simulink model "lab5_friccomp"  (Simulink 8.9)
settings: Solver=ode1  StartTime=0.0  StopTime=10  FixedStep=0.002  RelTol=1e-3  EnableMultiTasking=on
libraries: simulink x2, coecsllib x1, fricblocks x1
Description:
  | Real-Time Van der Pol Simulation
  | 
  | This demonstration shows a real-time version of the Simulink(R) Van der Pol
  | simulation demo. This model does not need any external signals, so it does
  | not need any data acquisition hardware or driver. This makes the model ideal
  | for first experiments with Real-Time Windows Target(TM), without need to
  | worry about proper I/O hardware configuration.
  | 
  | How to run this demo:
  | 
  |   1. Build the model using Tools -> Real-Time Workshop -> Build Model.
  |   2. Connect to the real-time code using Simulation -> Connect to target.
  |   3. Start the real-time execution using Simulation -> Start real-time code.
settings Model: Creator=Houska  LastModifiedBy=maherna4  SimulationMode=external  ExtModeTrigDuration=50000
settings DataIOCC: SignalLoggingName=logsOut
settings OptimizationCC: ExpressionDepthLimit=2147483647  InitFltsAndDblsToZero=on  EfficientMapNaN2IntZero=off  LifeSpan=auto
settings DebuggingCC: SignalResolutionControl=TryResolveAllWithWarning
settings HardwareCC: ProdBitPerPointer=64  ProdBitPerSizeT=64  ProdBitPerPtrDiffT=64  ProdLargestAtomicFloat=Float  ProdIntDivRoundTo=Zero  ProdEndianess=LittleEndian  ProdWordSize=64  ProdHWDeviceType=Intel->x86-64 (Windows64)  TargetBitPerLong=64  TargetBitPerPointer=64  TargetIntDivRoundTo=Zero  TargetEndianess=LittleEndian  TargetWordSize=64  TargetHWDeviceType=Intel->x86-64
settings RTWCC: SystemTargetFile=sldrt.tlc  TemplateMakefile=sldrt.tmf  Description=Simulink Desktop Real-Time  RTWCompilerOptimization=on
settings CodeAppCC: MaxIdLength=95
settings SimulinkDesktopRealTimeCC: TargetPreCompLibLocation=C:\MATLABR2017a\toolbox\sldrt\lib\win64  TargetLangStandard=C89/C90 (ANSI)  SupportVariableSizeSignals=off

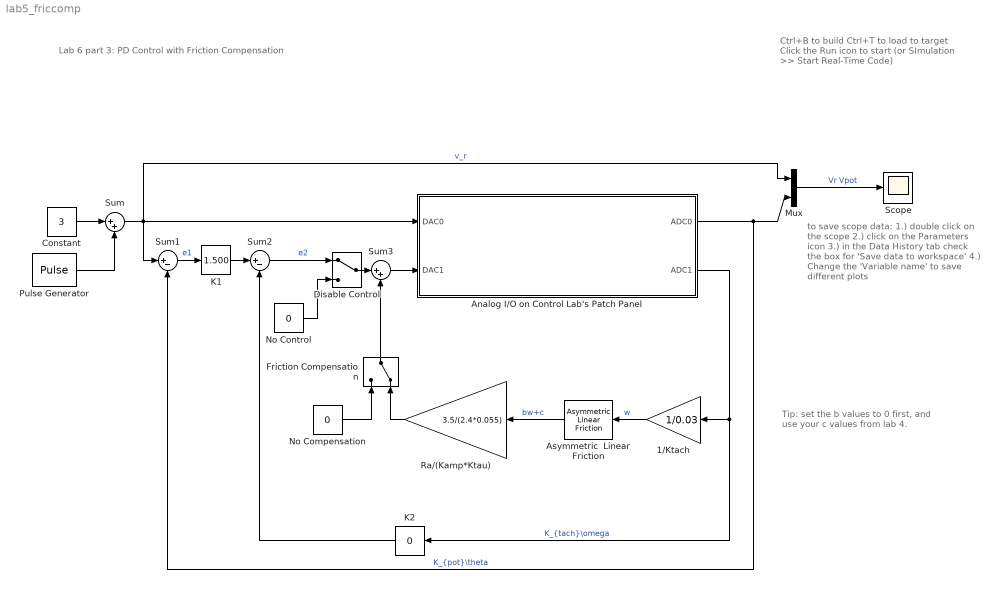
== system lab5_friccomp ==
  note: Lab 6 part 3: PD Control with Friction Compensation
  note: to save scope data:
      | 1.) double click on the scope
      | 2.) click on the Parameters icon
      | 3.) in the Data History tab check
      |  the box for 'Save data to workspace'
      | 4.) Change the 'Variable name'
      | to save different plots
  note: Ctrl+B to build
      | Ctrl+T to load to target
      | Click the Run icon to start
      | (or SImulation >> Start Real-Time Code)
  note: Tip: set the b values to 0 first, and
      | use your c values from lab 4.
  1/Ktach : Gain  Gain=1/0.03
  Analog I/O on Control Lab's Patch Panel : Subsystem  Description="Gives access to the Analog I/O ports on the patch panel used at UIUC's control labs.  Connects your digital controller to the analog I/O panel.  You can read in analog data through the ADCs (analog input) and output data using the DACs (analog output)"  mask(Analog I/O on Control Lab's Patch Panel){fixedstep=str2num(get_param(bdroot, 'FixedStep'))}
      mask prompts: fixedstep "Fixed-step size (fundamental sample time)"
      mask help: Gives access to the Analog I/O ports on the patch panel used at UIUC's control labs. This block connects your digital controller to the analog I/O panel. You can read in analog data from the two ADCs (analog input) and output data using the DACs (analog output)
      mask Help:
      | <h1 class="reftitle">Patch Panel: Analog I/O</h1>
      | 
      | <p>Gives access to the Analog I/O ports on the patch panel used at UIUC's control labs.  </p>
      | <h2>Description </h2><br>
      | 
      | This block connects your digital controller to the analog I/O panel.  You can read in analog data from the two ADCs (analog input) and output data using the DACs (analog output).
      | <p>
      | <p>
      | <hr>
      | Hint:  the controller and sensor inputs that Wincon uses are all Digital, while real-world signals (such as a Potentiometer voltage) are Analog.  If you want to output a control signal <i>u</i> to the real-world, you need to transform <i>u</i>  into an analog signal by using a <b>Digital to Analog Converter</b> (DAC).
      | <p>Similarly, to use the analog potentiometer voltage <i>V<sub>POT</sub></i> in your controller,  <i>V<sub>POT</sub></i> must first pass through an <b>Analog to Digital Converter</b> (ADC).
      | 
      | 
      | 
      | 
      |   <!-- Last updated: Thu April 5 18:42:05 EDT 2007-->
      |   <!-- Created by Aaron Becker-->
      mask Display:
      | image(imread('AnalogIO.bmp'))
      | disp('Patch Panel\nAnalog I/O')
      | color('white')
      | plot([0,0,4,4], [0,4,4,0])
      | color('red')
      | plot([0 0.5 0.5 0.76], [3.02 3.02 2.25 2.25])
      | color('green')
      | plot([0  1.3 1.3 1.15], [0.98  0.98 2.25 2.25])
      | color('blue')
      | plot([2.85 2.96 2.96  4.0], [1.15 1.15 3.02 3.02])
      | color('cyan')
      | plot([3.25 3.5 3.5 4.0], [1.15 1.15 0.98 0.98])
      | color('black')
      | port_label('input',1,'DAC0')
      | port_label('input',2,'DAC1')
      | port_label('output',1,'ADC0')
      | port_label('output',2,'ADC1')
  Asymmetric  Linear Friction : fricblocks/Asymmetric  Linear Friction  intercept1=(9.4E-3)*0.9  intercept2=-(1.2E-2)*0.9  slope1=(6.6E-5)*14.6*.5  slope2=(5E-5)*18*.5
  Constant : Constant  Value=3
  Disable Control : ManualSwitch
  Friction Compensation : ManualSwitch  CurrentSetting=0
  K1 : simulink/Math Operations/Slider Gain  gain=1.500  low=0  high=2
  K2 : simulink/Math Operations/Slider Gain  gain=0  low=0  high=10
  Mux : Mux  Inputs=2
  No Compensation : Constant  Value=0
  No Control : Constant  Value=0
  Pulse Generator : DiscretePulseGenerator  PulseType=Time based  Amplitude=2  PulseWidth=50
  Ra/(Kamp*Ktau) : Gain  Gain=3.5/(2.4*0.055)
  Scope : Scope
  Sum : Sum  Inputs=|++
  Sum1 : Sum  Inputs=|+-
  Sum2 : Sum  Inputs=|+-
  Sum3 : Sum  Inputs=|++
  wires:
  Constant/1 -> Sum/1
  Pulse Generator/1 -> Sum/2
  Sum/1 -> Analog I/O on Control Lab's Patch Panel/1(DAC0), Mux/1, Sum1/1  "v_r"
  Sum1/1 -> K1/1  "e1"
  K1/1 -> Sum2/1
  Analog I/O on Control Lab's Patch Panel/1(ADC0) -> Sum1/2, Mux/2  "K_{pot}\\theta"
  Analog I/O on Control Lab's Patch Panel/2(ADC1) -> K2/1, 1/Ktach/1  "K_{tach}\\omega"
  K2/1 -> Sum2/2
  Mux/1 -> Scope/1  "Vr Vpot"
  Sum2/1 -> Disable Control/1  "e2"
  No Control/1 -> Disable Control/2
  Disable Control/1 -> Sum3/1
  1/Ktach/1 -> Asymmetric  Linear Friction/1  "w"
  Friction Compensation/1 -> Sum3/2
  Asymmetric  Linear Friction/1 -> Ra/(Kamp*Ktau)/1  "bw+c"
  No Compensation/1 -> Friction Compensation/1
  Ra/(Kamp*Ktau)/1 -> Friction Compensation/2
  Sum3/1 -> Analog I/O on Control Lab's Patch Panel/2(DAC1)

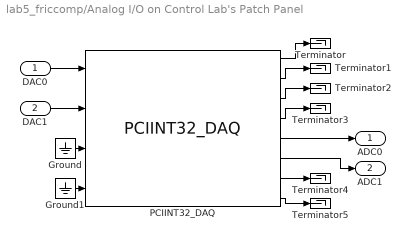
== system lab5_friccomp/Analog I/O on Control Lab's Patch Panel ==
  DAC0 : Inport
  DAC1 : Inport  Port=2
  Ground : Ground
  Ground1 : Ground
  PCIINT32_DAQ : coecsllib/Control Systems Lab Board Series/PCIINT32_DAQ  baddr2=findPCIint32BoardAddress3  sampleTime=str2num(get_param(bdroot, 'FixedStep'))
  Terminator{,1..5} (6 alike) : Terminator
  ADC0 : Outport
  ADC1 : Outport  Port=2
  wires:
  Ground1/1 -> PCIINT32_DAQ/4
  Ground/1 -> PCIINT32_DAQ/3
  PCIINT32_DAQ/8 -> Terminator5/1
  PCIINT32_DAQ/7 -> Terminator4/1
  PCIINT32_DAQ/4 -> Terminator3/1
  PCIINT32_DAQ/3 -> Terminator2/1
  PCIINT32_DAQ/2 -> Terminator1/1
  PCIINT32_DAQ/1 -> Terminator/1
  DAC0/1 -> PCIINT32_DAQ/1
  DAC1/1 -> PCIINT32_DAQ/2
  PCIINT32_DAQ/6 -> ADC1/1
  PCIINT32_DAQ/5 -> ADC0/1
